simulink model "EventAtTop"  (R2018b)
settings: Solver=FixedStepDiscrete  StartTime=0.0  StopTime=1  FixedStep=1  RelTol=1e-3
PreLoadFcn:
  | load test_data.mat;
model workspace (MATLAB code in the model file):
  | cmdLim = Simulink.Parameter;
  | cmdLim.Value = 15;
  | cmdLim.Description = 'Limit for controlling the maximum surface command angle.';
  | cmdLim.Min = 0;
  | cmdLim.Max = 90;
  | cmdLim.DocUnits = 'deg';
  | 
  | dispGain = Simulink.Parameter;
  | dispGain.Value = 0.75;
  | dispGain.Description = 'Gain applied to the displacement error.';
  | dispGain.Min = 0;
  | dispGain.Max = [];
  | dispGain.DocUnits = 'deg/sec/deg';
  | 
  | dispLim = Simulink.Parameter;
  | dispLim.Value = 30;
  | dispLim.Description = 'Limit for controlling the maximum commanded angle.';
  | dispLim.Min = 0;
  | dispLim.Max = 180;
  | dispLim.DocUnits = 'deg';
  | 
  | intGain = Simulink.Parameter;
  | intGain.Value = 0.5;
  | intGain.Description = 'Gain applied to the integral error.';
  | intGain.Min = 0;
  | intGain.Max = [];
  | intGain.DocUnits = 'deg/sec/deg/sec';
  | 
  | intLim = Simulink.Parameter;
  | intLim.Value = 5;
  | intLim.Description = 'Limit for controlling the maximum commanded angle.';
  | intLim.Min = 0;
  | intLim.Max = 90;
  | intLim.DocUnits = 'deg';
  | 
  | rateGain = Simulink.Parameter;
  | rateGain.Value = 2;
  | rateGain.Description = 'Gain applied to the rate error.';
  | rateGain.Min = 0;
  | rateGain.Max = [];
  | rateGain.DocUnits = 'deg/deg/sec';
  | 
  | rateLim = Simulink.Parameter;
  | rateLim.Value = 6;
  | rateLim.Description = 'Limit for controlling the maximum commanded angle.';
  | rateLim.Min = 0;
  | rateLim.Max = 180;
  | rateLim.DocUnits = 'deg/sec';
  | 
  | hdgGain = Simulink.Parameter;
  | hdgGain.Value = 0.015;
libraries: cfs_library x3
settings Model: RequirementInfo={} %GIDa_fe9045fd_0412_4b6e_8206_617cc20e6fde  FPTRunName=Active  TunableVars=K,initBus,initBus2  TunableVarsStorageClass=ExportedGlobal,ExportedGlobal,ExportedGlobal  TunableVarsTypeQualifier=,,  Creator=wstuart  LastModifiedBy=slentine
settings SolverCC: AutoInsertRateTranBlk=on
settings DataIOCC: SaveOutput=off  SignalLogging=off  DSMLogging=off  SaveTime=off
settings OptimizationCC: DefaultParameterBehavior=Inlined  UseDivisionForNetSlopeComputation=on  UseFloatMulNetSlope=on  EnhancedBackFolding=on  PassReuseOutputArgsAs=Individual arguments  EfficientFloat2IntCast=on  OptimizeBlockOrder=speed  DifferentSizesBufferReuse=on  OptimizationCustomize=off
settings DebuggingCC: ParameterTunabilityLossMsg=error  LibraryContextMissingDiagnostic=none  SFUnexpectedBacktrackingDiag=warning  SFNoUnconditionalDefaultTransitionDiag=warning  SFExecutionAtInitializationDiag=none
settings HardwareCC: ProdLongLongMode=on
settings SFSimCC: SimUseLocalCustomCode=off  MATLABDynamicMemAlloc=off
settings RTWCC: SystemTargetFile=cfs_ert.tlc  TLCOptions=-aCFE_GEN_STATE_TABLE=1  TemplateMakefile=ert_default_tmf  Description=NASA CFS Target File  GenerateReport=on  RetainRTWFile=on  RTWUseLocalCustomCode=off  BuildConfiguration=Faster Runs  IncludeHyperlinkInReport=on  LaunchReport=on  PortableWordSizes=on  GenerateTraceInfo=on  GenerateTraceReport=on  GenerateTraceReportSl=on  GenerateTraceReportSf=on  GenerateTraceReportEml=on
settings CodeAppCC: ForceParamTrailComments=on  IgnoreCustomStorageClasses=off  OperatorAnnotations=on  SimulinkDataObjDesc=on  SFDataObjDesc=on  InsertBlockDesc=on  EnableCustomComments=on
settings STFCustomTargetCC: TargetLangStandard=C99 (ISO)  MultiwordLength=256  GenerateSampleERTMain=on  CombineOutputUpdateFcns=on  ERTCustomFileBanners=on  SupportContinuousTime=off  SupportNonInlinedSFcns=off  RemoveResetFunc=on  MATLABClassNameForMDSCustomization=Simulink.SoftwareTarget.ERTCustomization  UseToolchainInfoCompliant=on  SystemTargetFile=cfs_ert.tlc
settings ERTTargetCC: TargetLangStandard=C99 (ISO)  GenerateSampleERTMain=on  ParMdlRefBuildCompliant=off  CompOptLevelCompliant=off  ConcurrentExecutionCompliant=off  ModelStepFunctionPrototypeControlCompliant=off  CPPClassGenCompliant=off  InlinedParameterPlacement=NonHierarchical  ERTCustomFileTemplate=cfs_interface.tlc
settings ConfigComp: CovScope=ReferencedModels  CovSaveName=covdata_rollAP  CovMetricSettings=dcmtrwe  CovHTMLOptions=-sRT=1 -aTS=1 -bRG=1 -bTC=1 -hTR=1 -nFC=0 -scm=1 -bcm=1 -xEv=0  CovSaveCumulativeToWorkspaceVar=on  CovSaveSingleToWorkspaceVar=on  CovCumulativeVarName=covCumulativeData_rollAP  CovReportOnPause=off  CovExternalEMLEnable=off  CovSFcnEnable=off

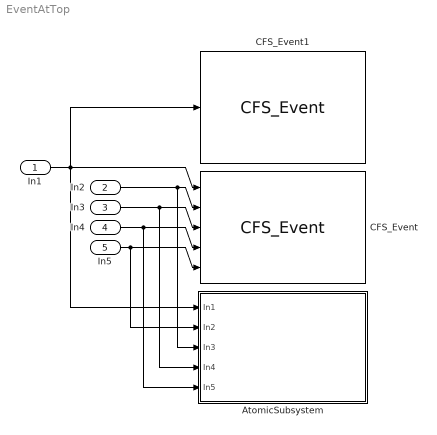
== system EventAtTop ==
  In1 : Inport  OutDataTypeStr=boolean
  In2 : Inport  Port=2  OutDataTypeStr=double
  In3 : Inport  Port=3  OutDataTypeStr=double
  In4 : Inport  Port=4  OutDataTypeStr=double
  In5 : Inport  Port=5  OutDataTypeStr=double
  AtomicSubsystem : Subsystem  TreatAsAtomicUnit=on
      settings: RTWFcnNameOpts=Use subsystem name  RTWFileNameOpts=Use subsystem name
  CFS_Event : cfs_library/CFS_Event  event_id=13  event_type=uint16(12)  event_mask=929  string_data='%f %e %e %f '  fmt_string=uint8(['Loc: %s, %f %e %e %f ' 0])  num_data_ports=4  block_sid=0
      settings: SourceProductName=CFS Blockset
  CFS_Event1 : cfs_library/CFS_Event  event_id=14  event_type=uint16(12)  event_mask=929  string_data=' '  fmt_string="uint8(['Loc: %s,  ' 0])"  num_data_ports=0  block_sid=0
      settings: SourceProductName=CFS Blockset
  wires:
  In1/1 -> AtomicSubsystem/1(In1), CFS_Event1/1, CFS_Event/1
  In2/1 -> AtomicSubsystem/3(In3), CFS_Event/2
  In3/1 -> AtomicSubsystem/4(In4), CFS_Event/3
  In4/1 -> AtomicSubsystem/5(In5), CFS_Event/4
  In5/1 -> AtomicSubsystem/2(In2), CFS_Event/5

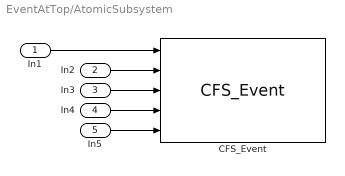
== system EventAtTop/AtomicSubsystem ==
  In1 : Inport  OutDataTypeStr=boolean
  In2 : Inport  Port=2  OutDataTypeStr=double
  In3 : Inport  Port=3  OutDataTypeStr=double
  In4 : Inport  Port=4  OutDataTypeStr=double
  In5 : Inport  Port=5  OutDataTypeStr=double
  CFS_Event : cfs_library/CFS_Event  event_id=15  event_type=uint16(12)  event_mask=929  string_data='%f %e %e %f '  fmt_string=uint8(['Loc: %s, %f %e %e %f ' 0])  num_data_ports=4  block_sid=0
      settings: SourceProductName=CFS Blockset
  wires:
  In1/1 -> CFS_Event/1
  In2/1 -> CFS_Event/2
  In3/1 -> CFS_Event/3
  In4/1 -> CFS_Event/4
  In5/1 -> CFS_Event/5
